simulink model "ConfiguredVirtualVehicleModelyaris"  (R2025b)
settings: configuration reference "VehicleVariable" (kept outside this file)
StartFcn:
  | %tic
StopFcn:
  | %toc
model workspace (MAT data in the model file):
  ExtDrvCmdsSwitch : Simulink.Parameter (value not decoded)
  ExtDrvRefSwitch : Simulink.Parameter (value not decoded)
  ExtEnvSwitch : Simulink.Parameter (value not decoded)
  ExtGndSwitch : Simulink.Parameter (value not decoded)
symbols that are objects in the model workspace (value not decoded): ExtDrvCmdsSwitch, ExtDrvRefSwitch, ExtEnvSwitch, ExtGndSwitch
undefined symbols (not defined in the file): AmbTemp, BaroPress, CurvGradRef, CurvRef, DCM, DriverAeroRes, DriverDrivelineRes, DriverInitialGear, DriverPreviewDist, DriverRollRes, DriverShiftTime, DriverTimeConst, DriverTractiveForce, EnvAbsPrs, EnvAirTemp, EnvGrvty, EnvNomFrictionScaling, EnvNominalGrade, EnvScnFrictionMap, EnvScnFrictionMapXBpts, EnvScnFrictionMapYBpts, EnvScnHeightMap, EnvScnHeightMapXBpts, EnvScnHeightMapYBpts, EnvWindVelX, EnvWindVelY, EnvWindVelZ, Gnd, Grade, HazzardCmd, HighBeamCmd, lambda_mux, LeftSignalCmd, LngRef, LowBeamCmd, LtrRef, PhiRef, PlntVehDstCGFrntAxl, PlntVehDstCGRearAxl, PlntVehInitLatPos, PlntVehInitLongPos, PlntVehInitPitchAng, PlntVehInitRollAng, PlntVehInitVertPos, PlntVehInitYawAng, PlntVehMass, PlntVehTrckWdth, PlntVehYawMomentInertia, PlntWhlLdRadiusFrnt, PlntWhlLdRadiusRear, RightSignalCmd, ScnCRRadius, Sim3dSensor, Wind, XRef, YRef, Z
libraries: simulink x28, autolibutils x8, autolibsharedcommon x7, vehdynlibscenariocommon x7, vehdynlibviscommon x4, vehdynlibdriver x2, sim3dgroundtruthsensorlib x2, sim3dlib x2, autolibshared x2, sim3dautolib x2, sl3dlib x1, sharedtransform x1
(part 3 of 6)

== system ConfiguredVirtualVehicleModelyaris/Visualization/External Output Routing ==
  VehFdbk : Inport
  Bus Assignment : BusAssignment  AssignedSignals=Driver.SteerFdbk,Driver.AccelFdbk,Driver.DecelFdbk,Driver.GearFdbk,Driver.IgnFdbk,Driveline.EngSpd,Driveline.TransGear,Body.InertFrm.Cg.Disp.X,Body.InertFrm.Cg.Disp.Y,Body.InertFrm.Cg.Disp.Z,Body.InertFrm.Cg.Vel.Xdot,Body.InertFrm.Cg.Vel.Ydot,Body.InertFrm.Cg.Vel.Zdot,Body.InertFrm.Cg.Ang.phi,Body.InertFrm.Cg.Ang.theta,Body.InertFrm.Cg.Ang.psi,Body.InertFrm.Geom.Disp.X,Body.InertFrm.Geom.Disp.Y,Body.InertFrm.Geom.Disp.Z,Body.InertFrm.Geom.Vel.Xdot,Body.InertFrm.Geom.Vel.Ydot,Body.InertFrm.Geom.Vel.Zdot,Body.BdyFrm.Cg.Vel.xdot,Body.BdyFrm.Cg.Vel.ydot,Body.BdyFrm.Cg.Vel.zdot,Body.BdyFrm.Cg.AngVel.p,Body.BdyFrm.Cg.AngVel.q,Body.BdyFrm.Cg.AngVel.r,Body.BdyFrm.Cg.Acc.ax,Body.BdyFrm.Cg.Acc.ay,Body.BdyFrm.Cg.Acc.az,Body.BdyFrm.Cg.Acc.xddot,Body.BdyFrm.Cg.Acc.yddot,Body.BdyFrm.Cg.Acc.zddot,Body.BdyFrm.Cg.AngAcc.pdot,Body.BdyFrm.Cg.AngAcc.qdot,Body.BdyFrm.Cg.AngAcc.rdot
  Bus Selector1 : BusSelector  OutputSignals=Driver.SteerFdbk,Driver.AccelFdbk,Driver.DecelFdbk,Driver.GearFdbk,Driver.IgnFdbk
  Bus Selector2 : BusSelector  OutputSignals=Body.InertFrm.Cg.Disp.X,Body.InertFrm.Cg.Disp.Y,Body.InertFrm.Cg.Disp.Z,Body.InertFrm.Cg.Vel.Xdot,Body.InertFrm.Cg.Vel.Ydot,Body.InertFrm.Cg.Vel.Zdot,Body.InertFrm.Cg.Ang.phi,Body.InertFrm.Cg.Ang.theta,Body.InertFrm.Cg.Ang.psi,Body.InertFrm.Geom.Disp.X,Body.InertFrm.Geom.Disp.Y,Body.InertFrm.Geom.Disp.Z,Body.InertFrm.Geom.Vel.Xdot,Body.InertFrm.Geom.Vel.Ydot,Body.InertFrm.Geom.Vel.Zdot,Body.BdyFrm.Cg.Vel.xdot,Body.BdyFrm.Cg.Vel.ydot,Body.BdyFrm.Cg.Vel.zdot,Body.BdyFrm.Cg.AngVel.p,Body.BdyFrm.Cg.AngVel.q,Body.BdyFrm.Cg.AngVel.r,Body.BdyFrm.Cg.Acc.ax,Body.BdyFrm.Cg.Acc.ay,Body.BdyFrm.Cg.Acc.az,Body.BdyFrm.Cg.Acc.xddot,Body.BdyFrm.Cg.Acc.yddot,Body.BdyFrm.Cg.Acc.zddot,Body.BdyFrm.Cg.AngAcc.pdot,Body.BdyFrm.Cg.AngAcc.qdot,Body.BdyFrm.Cg.AngAcc.rdot
  Bus Selector3 : BusSelector  OutputSignals=Engine.EngSpdOut,Trans.Info.Trans.TransGear
  Constant : Constant  Value=0  OutDataTypeStr=Bus: VVCVehFdbkBUS  SampleTime=-1
  Data Type Conversion : DataTypeConversion  SaturateOnIntegerOverflow=off  RndMeth=Floor
  Data Type Conversion1 : DataTypeConversion  SaturateOnIntegerOverflow=off  RndMeth=Floor
  Data Type Conversion2 : DataTypeConversion  SaturateOnIntegerOverflow=off  RndMeth=Floor
  Rate Transition : RateTransition  Integrity=off
  Rate Transition1 : RateTransition  Integrity=off
  Rate Transition2 : RateTransition  Integrity=off
  Unit Conversion{1..8} (8 alike) : UnitConversion
  ExtVehFdbk : Outport
  wires:
  Constant/1 -> Bus Assignment/1
  Bus Assignment/1 -> ExtVehFdbk/1
  Bus Selector1/1 -> Unit Conversion2/1  "<SteerFdbk>"
  Bus Selector1/2 -> Bus Assignment/3  "<AccelFdbk>"
  Bus Selector1/3 -> Bus Assignment/4  "<DecelFdbk>"
  Bus Selector1/4 -> Data Type Conversion1/1  "<GearFdbk>"
  Bus Selector1/5 -> Data Type Conversion2/1  "<IgnFdbk>"
  Bus Selector3/1 -> Unit Conversion1/1  "<EngSpdOut>"
  Bus Selector3/2 -> Data Type Conversion/1  "<TransGear>"
  Data Type Conversion/1 -> Bus Assignment/8
  Data Type Conversion1/1 -> Bus Assignment/5
  Data Type Conversion2/1 -> Bus Assignment/6
  Unit Conversion1/1 -> Bus Assignment/7
  Unit Conversion2/1 -> Bus Assignment/2
  Bus Selector2/1 -> Bus Assignment/9  "<X>"
  Bus Selector2/2 -> Bus Assignment/10  "<Y>"
  Bus Selector2/3 -> Bus Assignment/11  "<Z>"
  Bus Selector2/4 -> Bus Assignment/12  "<Xdot>"
  Bus Selector2/5 -> Bus Assignment/13  "<Ydot>"
  Bus Selector2/6 -> Bus Assignment/14  "<Zdot>"
  Bus Selector2/7 -> Unit Conversion6/1  "<phi>"
  Bus Selector2/8 -> Unit Conversion7/1  "<theta>"
  Bus Selector2/9 -> Unit Conversion8/1  "<psi>"
  Bus Selector2/10 -> Bus Assignment/18  "<X>"
  Bus Selector2/11 -> Bus Assignment/19  "<Y>"
  Bus Selector2/12 -> Bus Assignment/20  "<Z>"
  Bus Selector2/13 -> Bus Assignment/21  "<Xdot>"
  Bus Selector2/14 -> Bus Assignment/22  "<Ydot>"
  Bus Selector2/15 -> Bus Assignment/23  "<Zdot>"
  Bus Selector2/16 -> Bus Assignment/24  "<xdot>"
  Bus Selector2/17 -> Bus Assignment/25  "<ydot>"
  Bus Selector2/18 -> Bus Assignment/26  "<zdot>"
  Bus Selector2/19 -> Bus Assignment/27  "<p>"
  Bus Selector2/20 -> Bus Assignment/28  "<q>"
  Bus Selector2/21 -> Bus Assignment/29  "<r>"
  Bus Selector2/22 -> Unit Conversion3/1  "<ax>"
  Bus Selector2/23 -> Unit Conversion4/1  "<ay>"
  Bus Selector2/24 -> Unit Conversion5/1  "<az>"
  Bus Selector2/25 -> Bus Assignment/33  "<xddot>"
  Bus Selector2/26 -> Bus Assignment/34  "<yddot>"
  Bus Selector2/27 -> Bus Assignment/35  "<zddot>"
  Bus Selector2/28 -> Bus Assignment/36  "<pdot>"
  Bus Selector2/29 -> Bus Assignment/37  "<qdot>"
  Bus Selector2/30 -> Bus Assignment/38  "<rdot>"
  Unit Conversion3/1 -> Bus Assignment/30
  Unit Conversion4/1 -> Bus Assignment/31
  Unit Conversion5/1 -> Bus Assignment/32
  Unit Conversion6/1 -> Bus Assignment/15
  Unit Conversion7/1 -> Bus Assignment/16
  Unit Conversion8/1 -> Bus Assignment/17
  VehFdbk/1 -> Rate Transition/1, Rate Transition2/1, Rate Transition1/1
  Rate Transition/1 -> Bus Selector1/1
  Rate Transition1/1 -> Bus Selector3/1
  Rate Transition2/1 -> Bus Selector2/1

== system ConfiguredVirtualVehicleModelyaris/Visualization/ISO 15037-1:2006 ==
  VehFdbk : Inport
  Disabled : Subsystem  VariantControl=0
  Enabled : Subsystem  VariantControl=1

== system ConfiguredVirtualVehicleModelyaris/Visualization/Performance Calculations ==
  VehSpd : Inport
  FuelVolFlow : Inport  Port=2
  BattPwr : Inport  Port=3
  Add : Sum
  Divide : Product  Inputs=*/
  Divide1 : Product  Inputs=*/
  Divide2 : Product  Inputs=*/
  Integrator : Integrator
  Integrator1 : Integrator
  L/100 Km Calc : Product  Inputs=/*
  Product : Product
  Rate Transition3 : RateTransition  Deterministic=off
  Saturation : Saturate  UpperLimit=Inf  LowerLimit=0.001  ZeroCross=off
  Saturation1 : Saturate  UpperLimit=Inf  LowerLimit=1e-3  ZeroCross=off
  Signal Specification5 : SignalSpecification  Unit=m/s
  Sqrt : Sqrt
  US EPA kwh/USgal equivalent : Constant  Value=33.7
  US MPG Calc : Product  Inputs=*/
  Unit Conversion5 : UnitConversion
  m to 100Km : Gain  Gain=1/1000/100
  m to mile : Gain  Gain=0.000621371
  m^3 per gal : Gain  Gain=0.00378541
  m^3 to L : Gain  Gain=1000
  m^3 to US Gal : Gain  Gain=264.172
  s per h : Constant  Value=3600
  w per kw : Constant  Value=1000
  US MPG : Outport  VectorParamsAs1DForOutWhenUnconnected=off
  L/100Km : Outport  Port=2  VectorParamsAs1DForOutWhenUnconnected=off
  wires:
  m^3 to US Gal/1 -> Saturation1/1
  m^3 to L/1 -> L/100 Km Calc/2
  Integrator/1 -> m to mile/1, m to 100Km/1
  m to mile/1 -> US MPG Calc/1
  FuelVolFlow/1 -> Add/1
  Integrator1/1 -> m^3 to US Gal/1, m^3 to L/1
  Saturation/1 -> L/100 Km Calc/1
  m to 100Km/1 -> Saturation/1
  L/100 Km Calc/1 -> L/100Km/1  "L/100Km"
  US MPG Calc/1 -> Rate Transition3/1
  Saturation1/1 -> US MPG Calc/2
  Rate Transition3/1 -> US MPG/1  "US MPG"
  w per kw/1 -> Divide/2
  Divide/1 -> Divide2/1
  Divide2/1 -> Divide1/1
  s per h/1 -> Divide1/2
  Divide1/1 -> m^3 per gal/1
  Add/1 -> Integrator1/1
  m^3 per gal/1 -> Add/2
  US EPA kwh/USgal equivalent/1 -> Divide2/2
  BattPwr/1 -> Divide/1
  Sqrt/1 -> Integrator/1
  Product/1 -> Sqrt/1
  Signal Specification5/1 -> Product/2, Product/1
  Unit Conversion5/1 -> Signal Specification5/1
  VehSpd/1 -> Unit Conversion5/1

== system ConfiguredVirtualVehicleModelyaris/Visualization/Scope Type ==
  "VehFdbk " : Inport
  "Vis " : Inport  Port=2
  DLC : Subsystem  VariantControl=1
  None : Subsystem  VariantControl=0
  XYZ : Subsystem  VariantControl=2
  " Ref" : Outport  VectorParamsAs1DForOutWhenUnconnected=off

== system ConfiguredVirtualVehicleModelyaris/Visualization/Vehicle XY Plotter ==
  "VehFdbk " : Inport
  "Ref " : Inport  Port=2
  Disabled : Subsystem  VariantControl=2
  XY View : Subsystem  VariantControl=0
  XY View Ref : Subsystem  VariantControl=1
  XY View Ref with One-Axle Trailer : Subsystem  VariantControl=3

== system ConfiguredVirtualVehicleModelyaris/Driver Commands/Driver Commands/Dashboard Widgets ==
  note: Controls
  VehFdbk : Inport
  Hazards : LampBlock  LabelPosition=Hide  DefaultColor=[192.0, 192.0, 192.0]  Icon=Hazards
  High Beams : LampBlock  LabelPosition=Hide  DefaultColor=[192.0, 192.0, 192.0]  Icon=HighBeams
  Knob : KnobBlock  LabelPosition=Bottom  ScaleMin=-90  ScaleMax=90  TickInterval=30
  Low Beams : LampBlock  LabelPosition=Hide  DefaultColor=[192.0, 192.0, 192.0]  Icon=LowBeams
  Push Button : PushButtonBlock  ButtonText=Hazzard  ButtonType=Latch  Icon=Hazards  IconOnColor=[1.0, 0.0, 0.0]  IconOffColor=[0.50196078431372548, 0.50196078431372548, 0.50196078431372548]  IconColor=On  OffValue=0.000000
  Push Button1 : PushButtonBlock  ButtonText=Start / Stop  ButtonType=Latch  IconOnColor=[0.0, 1.0, 0.0]  IconOffColor=[0.0, 0.0, 0.0]  IconColor=On  OffValue=0.000000
  Rotary Switch : RotarySwitchBlock  LabelPosition=Bottom
  Rotary Switch1 : RotarySwitchBlock  LabelPosition=Bottom
  Rotary Switch2 : RotarySwitchBlock  LabelPosition=Bottom
  Slider : SliderBlock  LabelPosition=Bottom  ScaleMax=1  TickInterval=.2
  Slider1 : SliderBlock  LabelPosition=Bottom  ScaleMax=1  TickInterval=.2
  Turn Signal Left : LampBlock  LabelPosition=Hide  DefaultColor=[192.0, 192.0, 192.0]  Icon=TurnSignalLeft
  Turn Signal Right : LampBlock  LabelPosition=Hide  DefaultColor=[192.0, 192.0, 192.0]  Icon=TurnSignalRight
  Widget Sinks : Subsystem
  Widget Sources : Subsystem
  Driver : Outport  VectorParamsAs1DForOutWhenUnconnected=off
  wires:
  VehFdbk/1 -> Widget Sinks/1(VehFdbk)
  Widget Sources/1(Driver) -> Driver/1

== system ConfiguredVirtualVehicleModelyaris/Driver Commands/Driver Commands/Game Wheel Hardware ==
  VehFdbk : Inport
  Add : Sum  Inputs=-+
  Bus Creator1 : BusCreator  Inputs=6
  Compare To Zero : simulink/Logic and Bit Operations/Compare To Zero  relop=~=  OutDataTypeStr=boolean
  Constant : Constant  Value=false
  Constant1 : Constant
  Constant2 : Constant
  Cont LPF : autolibutils/Cont LPF  wc=10*2*pi  AbsoluteTolerance=auto  aMode=6
  Cont LPF1 : autolibutils/Cont LPF  wc=10*2*pi  AbsoluteTolerance=auto  aMode=6
  Dead Zone : DeadZone  LowerValue=0  UpperValue=.01  ZeroCross=off
  Demux1 : Demux  Outputs=2
  Gain : Gain  Gain=.5
  Game Wheel Input Requires Simulink 3D Animation Signal dimensions and scaling are hardware dependent : sl3dlib/Simulation 3D/Hardware Interface/Simulation 3D Joystick  Commented=on  joyid=1  adjustports=off  forcefeed=off
  Manual Switch : ManualSwitch  CurrentSetting=0
  OR : Logic  Operator=OR  IconShape=distinctive  AllPortsSameDT=off  OutDataTypeStr=boolean
  Paddle Shift : Subsystem
  Selector : Selector  InputPortWidth=8  IndexOptions=Index vector (dialog)  Indices=[1]  OutputSizes=1
  Selector1 : Selector  InputPortWidth=8  IndexOptions=Index vector (dialog)  Indices=[2 3]  OutputSizes=1
  Signal Specification : SignalSpecification  Unit=1
  Signal Specification1 : SignalSpecification  Unit=1
  Signal Specification2 : SignalSpecification  Unit=1
  Signal Specification3 : SignalSpecification  Unit=rad
  Stick Shift : Subsystem
  Switch : Switch  Criteria=u2 ~= 0  SaturateOnIntegerOverflow=off  InputSameDT=off
  Terminator : Terminator
  To Virtual Bus : SignalConversion  ConversionOutput=Virtual bus  OverrideOpt=off
  Unit Delay : UnitDelay  SampleTime=-1  HasFrameUpgradeWarning=on
  VVCLightsCmd : Constant  Value=0  OutDataTypeStr=Bus: VVCLightsCmdBUS  SampleTime=-1
  Wheel Angle Limit [rad] : Gain  Gain=2*2*pi
  Driver : Outport  VectorParamsAs1DForOutWhenUnconnected=off
  wires:
  Stick Shift/1(Gear) -> Manual Switch/2
  Paddle Shift/1(Gear) -> Manual Switch/1
  Game Wheel Input Requires Simulink 3D Animation Signal dimensions and scaling are hardware dependent/2 -> Paddle Shift/1(Buttons), Stick Shift/1(Buttons)
  Game Wheel Input Requires Simulink 3D Animation Signal dimensions and scaling are hardware dependent/1 -> Selector/1, Selector1/1
  To Virtual Bus/1 -> Bus Creator1/6  "LightsCmd"
  VVCLightsCmd/1 -> To Virtual Bus/1
  Constant1/1 -> Add/2
  Cont LPF/1 -> Wheel Angle Limit [rad]/1
  Demux1/1 -> Signal Specification/1
  Cont LPF1/1 -> Dead Zone/1
  Manual Switch/1 -> Signal Specification2/1
  Wheel Angle Limit [rad]/1 -> Signal Specification3/1
  Demux1/2 -> Signal Specification1/1
  Add/1 -> Gain/1
  Selector/1 -> Cont LPF/1
  Dead Zone/1 -> Demux1/1
  Gain/1 -> Cont LPF1/1
  Constant/1 -> Bus Creator1/5  "IgnSwtch"
  Signal Specification1/1 -> Bus Creator1/3  "DecelCmd"
  Signal Specification/1 -> Bus Creator1/2  "AccelCmd"
  VehFdbk/1 -> Terminator/1
  Bus Creator1/1 -> Driver/1
  Signal Specification3/1 -> Bus Creator1/1  "SteerCmd"
  Signal Specification2/1 -> Bus Creator1/4  "GearCmd"
  OR/1 -> Unit Delay/1, Switch/2
  Selector1/1 -> Switch/1, Compare To Zero/1
  Compare To Zero/1 -> OR/1
  Unit Delay/1 -> OR/2
  Switch/1 -> Add/1
  Constant2/1 -> Switch/3

== system ConfiguredVirtualVehicleModelyaris/Driver Commands/Driver Commands/Longitudinal Driver ==
  VehRef : Inport
  VehFdbk : Inport  Port=2
  Env : Inport  Port=3
  Bus Creator1 : BusCreator  Inputs=6
  Bus Selector1 : BusSelector  OutputSignals=DrvCmd.SteerCmd.SteerCmd,DrvRef.LngRef,DrvCmd.AccelCmd.EnblAccelCmd,DrvCmd.AccelCmd.AccelCmd,DrvCmd.AccelCmd.AccelHld,DrvCmd.AccelCmd.AccelZero,DrvCmd.DecelCmd.EnblDecelCmd,DrvCmd.DecelCmd.DecelCmd,DrvCmd.DecelCmd.DecelHld,DrvCmd.DecelCmd.DecelZero
  Constant : Constant  Value=false
  Hill Hold & Stop : Subsystem
  Longitudinal Driver : Subsystem  SystemSampleTime=.01  mask(Longitudinal Driver){extAccelOvr=on, extDecelOvr=on, extAccelHld=on, extDecelHld=on, extAccelZero=on, extDecelZero=on, cntrlType=Predictive, shftType=Reverse, Neutral, Drive, velUnits=m/s, gearOut=on, Kp=10, Ki=5, Kff=.1, Kg=0, VehVelVec=[0 100], KffVec=[.1 .1], KpVec=[10 10], KiVec=[5 5], KgVec=[0 0], m=PlntVehMass, Kpt=DriverTractiveForce, tau=DriverTimeConst, L=DriverPreviewDist, aR=DriverRollRes, bR=DriverDrivelineRes, cR=DriverAeroRes, g=EnvGrvty, vnom=5, Kaw=1, tauerr=.01, tauPt=2, GearInit=DriverInitialGear, tShift=DriverShiftTime, pdlVec=[0.1 0.4 0.5 0.9], upShftTbl=[-1 12.9375 26.4375 39.9375 51.18749999999999 62.4375 72.84375 83.25;-1 16.3125 29.8125 43.3125 54.5624 65.8125 76.78125 87.75;-1 19.6875 33.1875 46.68749999999999 57.9375 69.1875 80.71875 92.25;-1 33 52.5 77.25 100.5 138.75 161.875 185], dwnShftTbl=[1 9.5625 23.0625 36.5625 47.8125 59.0625 68.90625 78.75;1 12.9375 26.4375 39.9375 51.18749999999999 62.4375 72.84375 83.25;1 16.3125 29.8125 43.3125 54.562499 65.8125 76.78125 87.75;1 19.6875 33.1875 46.68749999999999 57.9375 69.1875 80.71875 92.25], tClutch=.5, tRev=.5, tPark=120, aMode=6, UpGearVec=[0  1  2  3  4  5  6  7], DownGearVec=[1  2  3  4  5  6  7  8]}
      mask prompts: extAccelOvr "autoblks_shared:autoblkLongitudinalDriver:blkPrm_extAccelOvr"; extDecelOvr "autoblks_shared:autoblkLongitudinalDriver:blkPrm_extDeccelOvr"; extAccelHld "autoblks_shared:autoblkLongitudinalDriver:blkPrm_extAccelHld"; extDecelHld "autoblks_shared:autoblkLongitudinalDriver:blkPrm_extDeccelHld"; extAccelZero "autoblks_shared:autoblkLongitudinalDriver:blkPrm_extAccelZero"; extDecelZero "autoblks_shared:autoblkLongitudinalDriver:blkPrm_extDeccelZero"; cntrlType "autoblks_shared:autoblkLongitudinalDriver:blkPrm_cntrlType"; shftType "autoblks_shared:autoblkLongitudinalDriver:blkPrm_shftType"; velUnits "autoblks_shared:autoblkLongitudinalDriver:blkPrm_velUnits"; gearOut "autoblks_shared:autoblkLongitudinalDriver:blkPrm_gearOut"; Kp "autoblks_shared:autoblkLongitudinalDriver:blkPrm_Kp"; Ki "autoblks_shared:autoblkLongitudinalDriver:blkPrm_Ki"; Kff "autoblks_shared:autoblkLongitudinalDriver:blkPrm_Kff"; Kg "autoblks_shared:autoblkLongitudinalDriver:blkPrm_Kg"; VehVelVec "autoblks_shared:autoblkLongitudinalDriver:blkPrm_VehVelVec"; KffVec "autoblks_shared:autoblkLongitudinalDriver:blkPrm_KffVec"; KpVec "autoblks_shared:autoblkLongitudinalDriver:blkPrm_KpVec"; KiVec "autoblks_shared:autoblkLongitudinalDriver:blkPrm_KiVec"; KgVec "autoblks_shared:autoblkLongitudinalDriver:blkPrm_KgVec"; m "autoblks_shared:autoblkLongitudinalDriver:blkPrm_m"; Kpt "autoblks_shared:autoblkLongitudinalDriver:blkPrm_Kpt"; tau "autoblks_shared:autoblkLongitudinalDriver:blkPrm_tau"; L "autoblks_shared:autoblkLongitudinalDriver:blkPrm_L"; aR "autoblks_shared:autoblkLongitudinalDriver:blkPrm_aR"; bR "autoblks_shared:autoblkLongitudinalDriver:blkPrm_bR"; cR "autoblks_shared:autoblkLongitudinalDriver:blkPrm_cR"; g "autoblks_shared:autoblkLongitudinalDriver:blkPrm_g"; vnom "autoblks_shared:autoblkLongitudinalDriver:blkPrm_vnom"; Kaw "autoblks_shared:autoblkLongitudinalDriver:blkPrm_Kaw"; tauerr "autoblks_shared:autoblkLongitudinalDriver:blkPrm_tauerr"; tauPt "autoblks_shared:autoblkLongitudinalDriver:blkPrm_tauPt"; GearInit "autoblks_shared:autoblkLongitudinalDriver:blkPrm_GearInit"; tShift "autoblks_shared:autoblkLongitudinalDriver:blkPrm_tShift"; pdlVec "autoblks_shared:autoblkLongitudinalDriver:blkPrm_pdlVec"; upShftTbl "autoblks_shared:autoblkLongitudinalDriver:blkPrm_upShftTbl"; dwnShftTbl "autoblks_shared:autoblkLongitudinalDriver:blkPrm_dwnShftTbl"; tClutch "autoblks_shared:autoblkLongitudinalDriver:blkPrm_tClutch"; tRev "autoblks_shared:autoblkLongitudinalDriver:blkPrm_tRev"; tPark "autoblks_shared:autoblkLongitudinalDriver:blkPrm_tPark"; UpGearVec "autoblks_shared:autoblkLongitudinalDriver:blkPrm_UpGearVec"; DownGearVec "autoblks_shared:autoblkLongitudinalDriver:blkPrm_DownGearVec"
      mask help: autoblks_shared:autoblkLongitudinalDriver:blkDesc
      mask init:
      | [~]=autosharedicon('autoliboperlong',gcb,0);
      mask Help: eval('autosharedhelp(''pbopmodlong'')');
      mask TypeOptions cntrlType: autoblks_shared:autoblkLongitudinalDriver:blkCmb_cntrlType_c1 | autoblks_shared:autoblkLongitudinalDriver:blkCmb_cntrlType_c2 | autoblks_shared:autoblkLongitudinalDriver:blkCmb_cntrlType_c3
      mask Callback cntrlType: [~]=autosharedicon('autoliboperlong',gcb,1);
      mask TypeOptions shftType: Longitudinal Driver/shftType
      mask Callback shftType: [~]=autosharedicon('autoliboperlong',gcb,1);
      mask TypeOptions velUnits: VelRef/Unit
      mask Callback velUnits: [~]=autosharedicon('autoliboperlong',gcb,1);
      mask DialogControl modeConfig Prompt: autoblks_shared:autoblkLongitudinalDriver:blkDlg_modeConfig
      mask DialogControl sigConfigPanel Prompt: autoblks_shared:autoblkLongitudinalDriver:blkDlg_sigConfigPanel
      mask DialogControl extAccelOvr Prompt: Accelerator override
      mask DialogControl extDecelOvr Prompt: Decelerator override
      mask DialogControl extAccelHld Prompt: Accelerator hold
      mask DialogControl extDecelHld Prompt: Decelerator hold
      mask DialogControl extAccelZero Prompt: Accelerator disable
      mask DialogControl extDecelZero Prompt: Decelerator disable
      mask DialogControl cntrlType Prompt: Control type, cntrlType:
      mask DialogControl shftType Prompt: Shift type, shftType:
      mask DialogControl velUnits Prompt: Reference and feedback units, velUnits [velUnits]:
      mask DialogControl gearOut Prompt: Output gear signal
      mask DialogControl CntrlParamPanel Prompt: autoblks_shared:autoblkLongitudinalDriver:blkDlg_CntrlParamPanel
      mask DialogControl PIParam Prompt: autoblks_shared:autoblkLongitudinalDriver:blkDlg_PIParam
      mask DialogControl Kp Prompt: Proportional gain, Kp []:
      mask DialogControl Ki Prompt: Integral gain, Ki []:
      mask DialogControl Kff Prompt: Velocity feed-forward, Kff []:
      mask DialogControl Kg Prompt: Grade angle feed-forward, Kg [1/deg]:
      mask DialogControl PISchedParam Prompt: autoblks_shared:autoblkLongitudinalDriver:blkDlg_PISchedParam
      mask DialogControl VehVelVec Prompt: Velocity gain breakpoints:
      mask DialogControl KffVec Prompt: Velocity feed-forward gain values, KffVec []:
      mask DialogControl KpVec Prompt: Proportional gain values, KpVec []:
      mask DialogControl KiVec Prompt: Integral gain values, KiVec []:
      mask DialogControl KgVec Prompt: Grade angle feed-forward values, KgVec [1/deg]:
      mask DialogControl PredParam Prompt: autoblks_shared:autoblkLongitudinalDriver:blkDlg_PredParam
      mask DialogControl m Prompt: Vehicle mass, m [kg]:
      mask DialogControl Kpt Prompt: Effective vehicle total tractive force, Kpt [N]:
      mask DialogControl tau Prompt: Driver response time, tau [s]:
      mask DialogControl L Prompt: Preview distance, L [m]:
      mask DialogControl aR Prompt: Rolling resistance coefficient, aR [N]:
      mask DialogControl bR Prompt: Rolling and driveline resistance coefficient, bR [N*s/m]:
      mask DialogControl cR Prompt: Aerodynamic drag coefficient, cR [N*s^2/m^2]:
      mask DialogControl g Prompt: Gravitational constant, g [m/s^2]:
      mask DialogControl vnom Prompt: Nominal speed, vnom [velUnits]:
      mask DialogControl Kaw Prompt: Anti-windup, Kaw []:
      mask DialogControl tauerr Prompt: Error filter time constant, tauerr [s]:
      mask DialogControl tauPt Prompt: Powertrain time constant, tauPt [s]:
      mask DialogControl shiftParamPanel Prompt: autoblks_shared:autoblkLongitudinalDriver:blkDlg_shiftParamPanel
      mask DialogControl GearInit Prompt: Initial gear, GearInit []:
      mask DialogControl tShift Prompt: Time required to shift, tShift [s]:
      mask DialogControl pdlVec Prompt: Up and down shift accelerator pedal positions, pdlVec []:
      mask DialogControl upShftTbl Prompt: Upshift velocity data table, upShftTbl [velUnits]:
      mask DialogControl dwnShftTbl Prompt: Downshift velocity data table, dwnShftTbl [velUnits]:
      mask DialogControl tClutch Prompt: Time required to shift, tClutch [s]:
      mask DialogControl tRev Prompt: Time required to engage reverse from neutral, tRev [s]:
      mask DialogControl tPark Prompt: Time required to engage park from neutral, tPark [s]:
      mask DialogControl UpGearVec Prompt: Upshift gear vector, UpGearVec []:
      mask DialogControl DownGearVec Prompt: Downshift gear vector, DownGearVec []:
      mask Display:
      | try
      |     IconInfo = autosharedicon('autoliboperlong', gcb, 4);
      | 
      |     image(IconInfo.image, IconInfo.position);
      | 
      |     for i = 1:numel(IconInfo.lconn)
      |         port_label('lconn', i, IconInfo.lconn{i})
      |     end
      | 
      |     for j = 1:numel(IconInfo.rconn)
      |         port_label('rconn', j, IconInfo.rconn{j})
      |     end
      | 
      |     for k = 1:numel(IconInfo.input)
      |         port_label('input', k, IconInfo.input{k})
      |     end
      | 
      |     for m = 1:numel(IconInfo.output)
      |         port_label('output', m, IconInfo.output{m})
      |     end
      | catch
      |     fprintf('Longitudinal \n Driver')
      | end
  Signal Specification : SignalSpecification  Unit=rad
  Terminator3 : Terminator
  To Nonvirtual Bus : SignalConversion  ConversionOutput=Virtual bus  OverrideOpt=off
  Unit Conversion : UnitConversion
  Unit Conversion1 : UnitConversion
  VVCLightsCmd : Constant  Value=0  OutDataTypeStr=Bus: VVCLightsCmdBUS  SampleTime=-1
  Driver : Outport  VectorParamsAs1DForOutWhenUnconnected=off
  wires:
  Signal Specification/1 -> Bus Creator1/1  "SteerCmd"
  To Nonvirtual Bus/1 -> Bus Creator1/6  "LightsCmd"
  VVCLightsCmd/1 -> To Nonvirtual Bus/1
  Hill Hold & Stop/6(Grade) -> Longitudinal Driver/11(Grade)
  Hill Hold & Stop/5(VelFdbk) -> Longitudinal Driver/10(VelFdbk)
  Bus Selector1/5 -> Longitudinal Driver/4(AccelHld)  "<AccelHld>"
  Unit Conversion1/1 -> Longitudinal Driver/1(VelRef), Hill Hold & Stop/1(LngRef)
  Hill Hold & Stop/4(DecelZero) -> Longitudinal Driver/9(DecelZero)
  Hill Hold & Stop/3(DecelHld) -> Longitudinal Driver/8(DecelHld)
  Env/1 -> Hill Hold & Stop/6(Env)
  Hill Hold & Stop/1(EnblDecelOvr) -> Longitudinal Driver/6(EnblDecelOvr)
  Hill Hold & Stop/2(DecelOvrCmd) -> Longitudinal Driver/7(DecelOvrCmd)
  Bus Selector1/10 -> Hill Hold & Stop/5(<DecelZero>)  "<DecelZero>"
  Bus Selector1/9 -> Hill Hold & Stop/4(<DecelHld>)  "<DecelHld>"
  Bus Selector1/8 -> Hill Hold & Stop/3(<DecelOvrCmd>)  "<DecelCmd>"
  Bus Selector1/7 -> Hill Hold & Stop/2(<EnblDecelCmd>)  "<EnblDecelCmd>"
  Bus Selector1/6 -> Longitudinal Driver/5(AccelZero)  "<AccelZero>"
  Bus Selector1/4 -> Longitudinal Driver/3(AccelOvrCmd)  "<AccelCmd>"
  Bus Selector1/3 -> Longitudinal Driver/2(EnblAccelOvr)  "<EnblAccelCmd>"
  Constant/1 -> Bus Creator1/5  "IgnSwtch"
  Bus Selector1/1 -> Unit Conversion/1  "<SteerCmd>"
  Longitudinal Driver/4(GearCmd) -> Bus Creator1/4  "GearCmd"
  Longitudinal Driver/2(AccelCmd) -> Bus Creator1/2  "AccelCmd"
  VehFdbk/1 -> Hill Hold & Stop/7(VehFdbk)
  VehRef/1 -> Bus Selector1/1
  Bus Selector1/2 -> Unit Conversion1/1  "<LngRef>"
  Longitudinal Driver/1(Info) -> Terminator3/1
  Longitudinal Driver/3(DecelCmd) -> Bus Creator1/3  "DecelCmd"
  Unit Conversion/1 -> Signal Specification/1
  Bus Creator1/1 -> Driver/1

== system ConfiguredVirtualVehicleModelyaris/Driver Commands/Driver Commands/No Driver ==
  VehRef : Inport
  VehFdbk : Inport  Port=2
  Env : Inport  Port=3
  Bus Creator1 : BusCreator  Inputs=6
  Bus Selector1 : BusSelector  OutputSignals=DrvCmd.SteerCmd.SteerCmd,DrvCmd.AccelCmd.AccelCmd,DrvCmd.DecelCmd.DecelCmd,DrvCmd.TransCmd.GearCmd,DrvCmd.IgnModeCmd,DrvCmd.LightsCmd
  Data Type Conversion : DataTypeConversion  SaturateOnIntegerOverflow=off  RndMeth=Floor
  Data Type Conversion1 : DataTypeConversion  SaturateOnIntegerOverflow=off  RndMeth=Floor
  Signal Specification{,1..3} (4 alike) : SignalSpecification  Unit=1
  Signal Specification4 : SignalSpecification  Unit=rad
  Terminator : Terminator
  Terminator1 : Terminator
  To Nonvirtual Bus : SignalConversion  ConversionOutput=Virtual bus  OverrideOpt=off
  Unit Conversion{,1..3} (4 alike) : UnitConversion
  Driver : Outport  VectorParamsAs1DForOutWhenUnconnected=off
  wires:
  Unit Conversion/1 -> Signal Specification4/1
  Data Type Conversion/1 -> Signal Specification3/1
  Unit Conversion3/1 -> Signal Specification2/1
  Unit Conversion2/1 -> Signal Specification1/1
  Unit Conversion1/1 -> Signal Specification/1
  Data Type Conversion1/1 -> Unit Conversion3/1
  Bus Selector1/5 -> Data Type Conversion/1  "<IgnModeCmd>"
  Bus Selector1/6 -> To Nonvirtual Bus/1  "<LightsCmd>"
  Bus Selector1/4 -> Data Type Conversion1/1  "<GearCmd>"
  Bus Selector1/3 -> Unit Conversion2/1  "<DecelCmd>"
  To Nonvirtual Bus/1 -> Bus Creator1/6  "LightsCmd"
  Env/1 -> Terminator1/1
  Signal Specification3/1 -> Bus Creator1/5  "IgnSwtch"
  Bus Selector1/1 -> Unit Conversion/1  "<SteerCmd>"
  Signal Specification2/1 -> Bus Creator1/4  "GearCmd"
  Signal Specification/1 -> Bus Creator1/2  "AccelCmd"
  VehFdbk/1 -> Terminator/1
  VehRef/1 -> Bus Selector1/1
  Bus Selector1/2 -> Unit Conversion1/1  "<AccelCmd>"
  Signal Specification1/1 -> Bus Creator1/3  "DecelCmd"
  Signal Specification4/1 -> Bus Creator1/1  "SteerCmd"
  Bus Creator1/1 -> Driver/1

== system ConfiguredVirtualVehicleModelyaris/Driver Commands/Driver Commands/Open Loop ==
  VehFdbk : Inport
  SteerCmd : Inport  Port=2
  AccelCmd : Inport  Port=3
  BrakeCmd : Inport  Port=4
  GearCmd : Inport  Port=5
  Bus Creator1 : BusCreator  Inputs=6
  Constant : Constant  Value=false
  Signal Specification : SignalSpecification  Unit=1
  Signal Specification1 : SignalSpecification  Unit=1
  Signal Specification2 : SignalSpecification  Unit=1
  Terminator : Terminator
  To Nonvirtual Bus : SignalConversion  ConversionOutput=Virtual bus  OverrideOpt=off
  Unit Conversion : UnitConversion
  VVCLightsCmd : Constant  Value=0  OutDataTypeStr=Bus: VVCLightsCmdBUS  SampleTime=-1
  Wheel Angle Limit * Steer Ratio : Gain  Gain=40*pi/180*18
  Driver : Outport  VectorParamsAs1DForOutWhenUnconnected=off
  wires:
  To Nonvirtual Bus/1 -> Bus Creator1/6  "LightsCmd"
  VVCLightsCmd/1 -> To Nonvirtual Bus/1
  Constant/1 -> Bus Creator1/5  "IgnSwtch"
  Signal Specification1/1 -> Bus Creator1/3  "DecelCmd"
  GearCmd/1 -> Signal Specification2/1
  Signal Specification/1 -> Bus Creator1/2  "AccelCmd"
  SteerCmd/1 -> Unit Conversion/1
  VehFdbk/1 -> Terminator/1
  AccelCmd/1 -> Signal Specification/1
  Unit Conversion/1 -> Wheel Angle Limit * Steer Ratio/1
  Bus Creator1/1 -> Driver/1
  Wheel Angle Limit * Steer Ratio/1 -> Bus Creator1/1  "SteerCmd"
  BrakeCmd/1 -> Signal Specification1/1
  Signal Specification2/1 -> Bus Creator1/4  "GearCmd"

== system ConfiguredVirtualVehicleModelyaris/Driver Commands/Driver Commands/Predictive Driver ==
  VehRef : Inport
  VehFdbk : Inport  Port=2
  Env : Inport  Port=3
  Bus Creator1 : BusCreator  Inputs=6
  Bus Selector : BusSelector  OutputSignals=Body.InertFrm.Cg.Disp.Y,Body.InertFrm.Cg.Vel.Ydot,Body.InertFrm.Cg.Ang.psi,Body.BdyFrm.Cg.AngVel.r
  Bus Selector1 : BusSelector  OutputSignals=DrvRef.LngRef,DrvRef.LtrRef,DrvCmd.SteerCmd.EnblSteerCmd,DrvCmd.SteerCmd.SteerCmd,DrvCmd.SteerCmd.SteerHld,DrvCmd.SteerCmd.SteerZero,DrvCmd.AccelCmd.EnblAccelCmd,DrvCmd.AccelCmd.AccelCmd,DrvCmd.AccelCmd.AccelHld,DrvCmd.AccelCmd.AccelZero,DrvCmd.DecelCmd.EnblDecelCmd,DrvCmd.DecelCmd.DecelCmd,DrvCmd.DecelCmd.DecelHld,DrvCmd.DecelCmd.DecelZero
  Constant : Constant  Value=false
  Hill Hold & Stop : Subsystem
  Linear Predictive Driver : vehdynlibdriver/Predictive Driver  extAccelOvr=on  extDecelOvr=on  extAccelHld=on  extDecelHld=on  extAccelZero=on  extDecelZero=on  extSteerOvr=on  extSteerHld=on  extSteerZero=on  cntrlType=Predictive  cntrlTypeLat=Predictive  shftType=Reverse, Neutral, Drive  coordMode=SAE J670 (Z-down)  refType=Reference pose  velUnits=m/s  angUnits=rad  gearOut=on  steerOut=on  Kp=3  Ki=1  Kff=1  Kg=0  VehVelVec=[0 100]  KffVec=[.1 .1]  KpVec=[10 10]  KiVec=[5 5]  KgVec=[0 0]  vnom=5  Kaw=1  tauerr=.075  tau=DriverTimeConst  L=DriverPreviewDist  Kpt=DriverTractiveForce  aR=DriverRollRes  bR=DriverDrivelineRes  cR=DriverAeroRes  g=EnvGrvty  vecPose=off  dynamMode=off  PositionGainF=2.5  PositionGainR=2.5  YawRateGain=.2  DelayGain=.2  enableDrift=off  BetaRef=10  KpBeta=1  KpDrift=1  KdDrift=1  KpPsi=1  KOmega=.1  tOmega=.1  a=PlntVehDstCGFrntAxl  b=PlntVehDstCGRearAxl  m=PlntVehMass  Cy_f=DriverFrontCornerStiff  Cy_r=DriverRearCornerStiff  I=PlntVehYawMomentInertia  Ksteer=PlntSteerRatio  theta=DriverWheelRange  Idl=1  Re=PlntWhlLdRadius  lambda_mu=1  GearInit=DriverInitialGear  tShift=DriverShiftTime  pdlVec=[0.1 0.4 0.5 0.9]  upShftTbl=[-1 12.9375 26.4375 39.9375 51.18749999999999 62.4375 72.84375 83.25;-1 16.3125 29.8125 43.3125 54.5624 65.8125 76.78125 87.75;-1 19.6875 33.1875 46.68749999999999 57.9375 69.1875 80.71875 92.25;-1 33 52.5 77.25 100.5 138.75 161.875 185]  dwnShftTbl=[-1 12.9375 26.4375 39.9375 51.18749999999999 62.4375 72.84375 83.25;-1 16.3125 29.8125 43.3125 54.5624 65.8125 76.78125 87.75;-1 19.6875 33.1875 46.68749999999999 57.9375 69.1875 80.71875 92.25;-1 33 52.5 77.25 100.5 138.75 161.875 185]  tClutch=.5  tRev=.5  tPark=120  UpGearVec="[0  1  2  3  4  5  6  7]"  DownGearVec="[1  2  3  4  5  6  7  8]"  aMode=2
  Terminator : Terminator
  To Nonvirtual Bus : SignalConversion  ConversionOutput=Virtual bus  OverrideOpt=off
  Unit Conversion : UnitConversion
  VVCLightsCmd : Constant  Value=0  OutDataTypeStr=Bus: VVCLightsCmdBUS  SampleTime=-1
  Driver : Outport  VectorParamsAs1DForOutWhenUnconnected=off
  wires:
  Bus Selector1/14 -> Hill Hold & Stop/5(<DecelZero>)  "<DecelZero>"
  To Nonvirtual Bus/1 -> Bus Creator1/6  "LightsCmd"
  VVCLightsCmd/1 -> To Nonvirtual Bus/1
  Unit Conversion/1 -> Linear Predictive Driver/1, Hill Hold & Stop/1(LngRef)
  Hill Hold & Stop/1(EnblDecelOvr) -> Linear Predictive Driver/11
  Hill Hold & Stop/2(DecelOvrCmd) -> Linear Predictive Driver/12
  Hill Hold & Stop/3(DecelHld) -> Linear Predictive Driver/13
  Hill Hold & Stop/4(DecelZero) -> Linear Predictive Driver/14
  Hill Hold & Stop/6(VelFdbk) -> Linear Predictive Driver/16
  Hill Hold & Stop/5(Grade) -> Linear Predictive Driver/15
  Env/1 -> Hill Hold & Stop/6(Env)
  Bus Selector1/13 -> Hill Hold & Stop/4(<DecelHld>)  "<DecelHld>"
  Bus Selector1/12 -> Hill Hold & Stop/3(<DecelOvrCmd>)  "<DecelCmd>"
  Bus Selector1/11 -> Hill Hold & Stop/2(<EnblDecelCmd>)  "<EnblDecelCmd>"
  Bus Selector1/9 -> Linear Predictive Driver/9  "<AccelHld>"
  Bus Selector1/8 -> Linear Predictive Driver/8  "<AccelCmd>"
  Bus Selector1/7 -> Linear Predictive Driver/7  "<EnblAccelCmd>"
  Bus Selector1/6 -> Linear Predictive Driver/6  "<SteerZero>"
  Bus Selector1/5 -> Linear Predictive Driver/5  "<SteerHld>"
  Bus Selector1/4 -> Linear Predictive Driver/4  "<SteerCmd>"
  Bus Selector1/3 -> Linear Predictive Driver/3  "<EnblSteerCmd>"
  Constant/1 -> Bus Creator1/5  "IgnSwtch"
  Linear Predictive Driver/5 -> Bus Creator1/4  "GearCmd"
  Linear Predictive Driver/4 -> Bus Creator1/3  "DecelCmd"
  Linear Predictive Driver/2 -> Bus Creator1/1  "SteerCmd"
  Bus Selector1/1 -> Unit Conversion/1  "<LngRef>"
  VehRef/1 -> Bus Selector1/1
  Bus Selector/4 -> Linear Predictive Driver/20  "<r>"
  Bus Selector1/2 -> Linear Predictive Driver/2  "<LtrRef>"
  VehFdbk/1 -> Bus Selector/1, Hill Hold & Stop/7(VehFdbk)
  Bus Selector/3 -> Linear Predictive Driver/19  "<psi>"
  Linear Predictive Driver/1 -> Terminator/1
  Bus Creator1/1 -> Driver/1
  Bus Selector1/10 -> Linear Predictive Driver/10  "<AccelZero>"
  Bus Selector/1 -> Linear Predictive Driver/17  "<Y>"
  Linear Predictive Driver/3 -> Bus Creator1/2  "AccelCmd"
  Bus Selector/2 -> Linear Predictive Driver/18  "<Ydot>"

== system ConfiguredVirtualVehicleModelyaris/Driver Commands/Driver Commands/Predictive Stanley Driver ==
  VehRef : Inport
  VehFdbk : Inport  Port=2
  Env : Inport  Port=3
  Bus Creator1 : BusCreator  Inputs=6
  Bus Selector : BusSelector  OutputSignals=Body.InertFrm.Cg.Disp.X,Body.InertFrm.Cg.Disp.Y,Body.InertFrm.Cg.Ang.psi,Body.BdyFrm.Cg.AngVel.r
  Bus Selector1 : BusSelector  OutputSignals=DrvRef.LngRef,DrvRef.XRef,DrvRef.YRef,DrvRef.PhiRef,DrvCmd.SteerCmd.EnblSteerCmd,DrvCmd.SteerCmd.SteerCmd,DrvCmd.SteerCmd.SteerHld,DrvCmd.SteerCmd.SteerZero,DrvCmd.AccelCmd.EnblAccelCmd,DrvCmd.AccelCmd.AccelCmd,DrvCmd.AccelCmd.AccelHld,DrvCmd.AccelCmd.AccelZero,DrvCmd.DecelCmd.EnblDecelCmd,DrvCmd.DecelCmd.DecelCmd,DrvCmd.DecelCmd.DecelHld,DrvCmd.DecelCmd.DecelZero,DrvRef.CurvRef
  Constant : Constant  Value=false
  Hill Hold & Stop : Subsystem
  Linear Predictive Driver : vehdynlibdriver/Predictive Driver  extAccelOvr=on  extDecelOvr=on  extAccelHld=on  extDecelHld=on  extAccelZero=on  extDecelZero=on  extSteerOvr=on  extSteerHld=on  extSteerZero=on  cntrlType=Predictive  cntrlTypeLat=Stanley  shftType=Reverse, Neutral, Drive  coordMode=SAE J670 (Z-down)  refType=Reference pose  velUnits=m/s  angUnits=rad  gearOut=on  steerOut=on  Kp=3  Ki=1  Kff=1  Kg=0  VehVelVec=[0 100]  KffVec=[.1 .1]  KpVec=[10 10]  KiVec=[5 5]  KgVec=[0 0]  vnom=5  Kaw=1  tauerr=.075  tau=DriverTimeConst  L=DriverPreviewDist  Kpt=DriverTractiveForce  aR=DriverRollRes  bR=DriverDrivelineRes  cR=DriverAeroRes  g=EnvGrvty  vecPose=off  dynamMode=on  PositionGainF=DriverPositionGainF  PositionGainR=DriverPositionGainR  YawRateGain=DriverYawRateGain  DelayGain=DriverDelayGain  enableDrift=off  BetaRef=10  KpBeta=1  KpDrift=1  KdDrift=1  KpPsi=1  KOmega=.1  tOmega=.1  a=PlntVehDstCGFrntAxl  b=PlntVehDstCGRearAxl  m=PlntVehMass  Cy_f=DriverFrontCornerStiff  Cy_r=DriverRearCornerStiff  I=PlntVehYawMomentInertia  Ksteer=PlntSteerRatio  theta=DriverWheelRange  Idl=1  Re=PlntWhlLdRadius  lambda_mu=1  GearInit=DriverInitialGear  tShift=DriverShiftTime  pdlVec=[0.1 0.4 0.5 0.9]  upShftTbl=[-1 12.9375 26.4375 39.9375 51.18749999999999 62.4375 72.84375 83.25;-1 16.3125 29.8125 43.3125 54.5624 65.8125 76.78125 87.75;-1 19.6875 33.1875 46.68749999999999 57.9375 69.1875 80.71875 92.25;-1 33 52.5 77.25 100.5 138.75 161.875 185]  dwnShftTbl=[-1 12.9375 26.4375 39.9375 51.18749999999999 62.4375 72.84375 83.25;-1 16.3125 29.8125 43.3125 54.5624 65.8125 76.78125 87.75;-1 19.6875 33.1875 46.68749999999999 57.9375 69.1875 80.71875 92.25;-1 33 52.5 77.25 100.5 138.75 161.875 185]  tClutch=.5  tRev=.5  tPark=120  UpGearVec="[0  1  2  3  4  5  6  7]"  DownGearVec="[1  2  3  4  5  6  7  8]"  aMode=2
  Terminator : Terminator
  To Nonvirtual Bus : SignalConversion  ConversionOutput=Virtual bus  OverrideOpt=off
  Unit Conversion : UnitConversion
  VVCLightsCmd : Constant  Value=0  OutDataTypeStr=Bus: VVCLightsCmdBUS  SampleTime=-1
  Driver : Outport  VectorParamsAs1DForOutWhenUnconnected=off
  wires:
  Bus Selector1/13 -> Hill Hold & Stop/2(<EnblDecelCmd>)  "<EnblDecelCmd>"
  Bus Selector1/14 -> Hill Hold & Stop/3(<DecelOvrCmd>)  "<DecelCmd>"
  Bus Selector1/15 -> Hill Hold & Stop/4(<DecelHld>)  "<DecelHld>"
  Bus Selector1/16 -> Hill Hold & Stop/5(<DecelZero>)  "<DecelZero>"
  Bus Selector1/17 -> Hill Hold & Stop/6(<CurvRef>)  "<CurvRef>"
  Bus Selector1/12 -> Linear Predictive Driver/12  "<AccelZero>"
  Bus Selector/1 -> Linear Predictive Driver/20  "<X>"
  Bus Selector/2 -> Linear Predictive Driver/21  "<Y>"
  Bus Selector/3 -> Linear Predictive Driver/22  "<psi>"
  Bus Selector1/2 -> Linear Predictive Driver/2  "<XRef>"
  Bus Selector1/3 -> Linear Predictive Driver/3  "<YRef>"
  Bus Selector1/4 -> Linear Predictive Driver/4  "<PhiRef>"
  Bus Selector1/5 -> Linear Predictive Driver/5  "<EnblSteerCmd>"
  Bus Selector1/10 -> Linear Predictive Driver/10  "<AccelCmd>"
  Bus Selector1/6 -> Linear Predictive Driver/6  "<SteerCmd>"
  Bus Selector1/9 -> Linear Predictive Driver/9  "<EnblAccelCmd>"
  Bus Selector1/7 -> Linear Predictive Driver/7  "<SteerHld>"
  Bus Selector1/8 -> Linear Predictive Driver/8  "<SteerZero>"
  To Nonvirtual Bus/1 -> Bus Creator1/6  "LightsCmd"
  VVCLightsCmd/1 -> To Nonvirtual Bus/1
  Hill Hold & Stop/6(CurvRef) -> Linear Predictive Driver/18
  Hill Hold & Stop/5(Grade) -> Linear Predictive Driver/17
  Bus Selector/4 -> Linear Predictive Driver/23  "<r>"
  Linear Predictive Driver/3 -> Bus Creator1/2  "AccelCmd"
  Bus Creator1/1 -> Driver/1
  Linear Predictive Driver/1 -> Terminator/1
  VehFdbk/1 -> Bus Selector/1, Hill Hold & Stop/8(VehFdbk)
  VehRef/1 -> Bus Selector1/1
  Bus Selector1/1 -> Unit Conversion/1  "<LngRef>"
  Linear Predictive Driver/2 -> Bus Creator1/1  "SteerCmd"
  Linear Predictive Driver/4 -> Bus Creator1/3  "DecelCmd"
  Linear Predictive Driver/5 -> Bus Creator1/4  "GearCmd"
  Constant/1 -> Bus Creator1/5  "IgnSwtch"
  Bus Selector1/11 -> Linear Predictive Driver/11  "<AccelHld>"
  Env/1 -> Hill Hold & Stop/7(Env)
  Hill Hold & Stop/7(VelFdbk) -> Linear Predictive Driver/19
  Hill Hold & Stop/4(DecelZero) -> Linear Predictive Driver/16
  Hill Hold & Stop/3(DecelHld) -> Linear Predictive Driver/15
  Hill Hold & Stop/2(DecelOvrCmd) -> Linear Predictive Driver/14
  Hill Hold & Stop/1(EnblDecelOvr) -> Linear Predictive Driver/13
  Unit Conversion/1 -> Linear Predictive Driver/1, Hill Hold & Stop/1(LngRef)

== system ConfiguredVirtualVehicleModelyaris/Environment/Ground Feedback/3D Engine ==
  WheelFdbk : Inport
  3D Engine Source : Subsystem  Variant=on  VariantControl=Choice  mask(Terrain Source){terrType=Single point}
      mask prompts: terrType "Terrain feedback type:"
      mask help:
      | This variant subsystem provides the option for:
      | - a single point of contact for each wheel with minimal post-processing ideal for smooth surfaces and maximum run-time performance.
      | - multiple points of contact per wheel which may be used when interested in non-smooth terrain at a higher computational cost and requires Vehicle Dynamics Blockset.
      mask TypeOptions terrType: Single point | Multiple points
  Z : Outport  VectorParamsAs1DForOutWhenUnconnected=off
  DCM : Outport  Port=2  VectorParamsAs1DForOutWhenUnconnected=off
  wires:
  WheelFdbk/1 -> 3D Engine Source/1(WheelFdbk)
  3D Engine Source/1(z) -> Z/1
  3D Engine Source/2(DCM) -> DCM/1

== system ConfiguredVirtualVehicleModelyaris/Environment/Ground Feedback/Constant ==
  Bus Creator : BusCreator  Inputs=4
  Constant1 : Constant  Value=zeros(4,1)
  Constant2 : Constant  Value=repmat(eye(3),1,1,4)  SampleTime=-1
  Demux : Demux
  Signal Specification : SignalSpecification  Unit=m
  Z : Outport  VectorParamsAs1DForOutWhenUnconnected=off
  DCM : Outport  Port=2  VectorParamsAs1DForOutWhenUnconnected=off
  wires:
  Constant1/1 -> Signal Specification/1
  Signal Specification/1 -> Demux/1
  Demux/4 -> Bus Creator/4  "G_RR_z"
  Demux/1 -> Bus Creator/1  "G_FL_z"
  Demux/3 -> Bus Creator/3  "G_RL_z"
  Demux/2 -> Bus Creator/2  "G_FR_z"
  Bus Creator/1 -> Z/1  "z"
  Constant2/1 -> DCM/1  "DCM"

== system ConfiguredVirtualVehicleModelyaris/Environment/Ground Feedback/Height Map ==
  InertFrm : Inport
  "2D Lookup Tbl for Elevation, Z" : Subsystem  TreatAsAtomicUnit=on
      mask init:
      | [~]=vehdynicon('vehdynblk',gcb);
  Bus Creator : BusCreator  Inputs=4
  Bus Selector : BusSelector  OutputSignals=FrntAxl.Lft.Disp.X,FrntAxl.Rght.Disp.X,RearAxl.Lft.Disp.X,RearAxl.Rght.Disp.X
  Bus Selector1 : BusSelector  OutputSignals=FrntAxl.Lft.Disp.Y,FrntAxl.Rght.Disp.Y,RearAxl.Lft.Disp.Y,RearAxl.Rght.Disp.Y
  Constant2 : Constant  Value=repmat(eye(3),1,1,4)  SampleTime=-1
  Demux : Demux
  Signal Specification : SignalSpecification  Unit=m
  Wheel Coordinates : Subsystem
  Z : Outport
  DCM : Outport  Port=2
  wires:
  "2D Lookup Tbl for Elevation, Z"/1(Z) -> Signal Specification/1
  Bus Selector1/4 -> Wheel Coordinates/8(RearAxlRghtY)  "<Y>"
  Bus Selector1/3 -> Wheel Coordinates/7(RearAxlLftY)  "<Y>"
  Bus Selector/1 -> Wheel Coordinates/1(FrntAxlLftX)  "<X>"
  Bus Selector/2 -> Wheel Coordinates/2(FrntAxlRghtX)  "<X>"
  Bus Selector1/2 -> Wheel Coordinates/6(FrntAxlRghtY)  "<Y>"
  Bus Selector/4 -> Wheel Coordinates/4(RearAxlRghtX)  "<X>"
  Bus Selector/3 -> Wheel Coordinates/3(RearAxlLftX)  "<X>"
  Bus Selector1/1 -> Wheel Coordinates/5(FrntAxlLftY)  "<Y>"
  Wheel Coordinates/2(YWhl) -> "2D Lookup Tbl for Elevation, Z"/2(YWhl)
  Wheel Coordinates/1(XWhl) -> "2D Lookup Tbl for Elevation, Z"/1(XWhl)
  InertFrm/1 -> Bus Selector1/1, Bus Selector/1
  Demux/2 -> Bus Creator/2  "G_FR_z"
  Demux/1 -> Bus Creator/1  "G_FL_z"
  Demux/4 -> Bus Creator/4  "G_RR_z"
  Demux/3 -> Bus Creator/3  "G_RL_z"
  Bus Creator/1 -> Z/1  "z"
  Signal Specification/1 -> Demux/1
  Constant2/1 -> DCM/1  "DCM"

== system ConfiguredVirtualVehicleModelyaris/Environment/Ground Feedback/Ideal Inclined Plane ==
  InertFrm : Inport
  Bus Creator : BusCreator  Inputs=4
  Bus Selector : BusSelector  OutputSignals=FrntAxl.Lft.Disp.X,FrntAxl.Rght.Disp.X,RearAxl.Lft.Disp.X,RearAxl.Rght.Disp.X
  Bus Selector1 : BusSelector  OutputSignals=FrntAxl.Lft.Disp.Y,FrntAxl.Rght.Disp.Y,RearAxl.Lft.Disp.Y,RearAxl.Rght.Disp.Y
  Demux : Demux
  Ideal Inclined Plane : Subsystem  mask(Ideal Plane Elevation Generator){phi_o=0, theta_o=0, Z_o=0, psi_o=-PlntVehInitYawAng, phi_est=0, theta_est=0, Z_est=5, plane3D=off, planeX=200, planeY=200}
      mask prompts: phi_o "Initial plane bank angle (about global X axis) [rad]:"; theta_o "Initial plane pitch angle (about global Y axis)  [rad]:"; Z_o "Initial plane elevation (at [0,0,0]) [m]"; psi_o "Initial vehicle yaw angle (about global Z axis) [rad]:"; phi_est "Estimated initial vehicle roll angle [rad]:"; theta_est "Estimated initial vehicle pitch angle [rad]:"; Z_est "Estimated initial vehicle elevation [m]"; plane3D "Enable 3D visualization of plane. Requires the Simulink 3D Animation and the 3D visualization enabled (in the Visualization subsystem). The Empty Scene is recommended when activated."; planeX "Total plane length (in X dimension) [m]:"; planeY "Total plane width (in Y dimension) [m]:"
      mask help:
      | This block accepts time varying bank and pitch angles for an idealized planar surface centered at the global origin (Z+up).
      | The plane roll or bank angle, phi, is about the X axis and pitch angle, theta (negative grade), is about the Y axis.
      | A static vertical offset, Z_o, is also permited.
      | Based on the initial plane angles and vertical offset and vehicle pose, estimates of the initial vehicle roll and pitch are calculated (in the vehicle Z+ down frame). These values can be optionally used to udpate the sldds.
      | Caution should be used to esnure the input signals and initial parameters are consistent at initialzation time.
      | If Simulink 3D Animation is available, the visualization will also include a planar checkerboard surface (changing the default scene may be desired in the Visualization subsystem).
      mask init:
      | vehdynicon('vehdynlibzplane',gcb,0,[]);
      mask Callback plane3D: vehdynicon('vehdynlibzplane',gcb,1,[]);
      mask DialogControl initParams Prompt: Setup Parameters
      mask DialogControl slddUpdate Prompt: Vehicle Pose Estimates
      mask DialogControl updateSLDD Prompt: Update data dictionary with initial roll, pitch and yaw estimates
      mask DialogControl updateSLDD Callback: vehdynicon('vehdynlibzplane',gcb,2,'VirtualVehicleTemplate.sldd');
      mask DialogControl sim3d Prompt: Visualization Options
  Rate Limiter : RateLimiter  RisingSlewLimit=10  FallingSlewLimit=-10  SampleTimeMode=inherited
  Rate Limiter1 : RateLimiter  RisingSlewLimit=10  FallingSlewLimit=-10  SampleTimeMode=inherited
  Signal Specification : SignalSpecification  Unit=m
  Signal Specification1 : SignalSpecification  Unit=deg
  Signal Specification2 : SignalSpecification  Unit=deg
  Slider : SliderBlock  ScaleMin=-30  ScaleMax=30
  Slider1 : SliderBlock  ScaleMin=-30  ScaleMax=30
  Unit Conversion : UnitConversion
  Unit Conversion1 : UnitConversion
  Vector Concatenate : Concatenate  NumInputs=4  Mode=Multidimensional array  ConcatenateDimension=3
  Wheel Coordinates : Subsystem
  Z+up : UnaryMinus
  phiPlane : Constant  Value=0
  thetaPlane : Constant  Value=0
  Z : Outport
  DCM : Outport  Port=2
  wires:
  Ideal Inclined Plane/2(DCM) -> Vector Concatenate/1, Vector Concatenate/2, Vector Concatenate/4, Vector Concatenate/3  "DCM"
  Signal Specification/1 -> Demux/1
  Bus Creator/1 -> Z/1  "z"
  Demux/3 -> Bus Creator/3  "G_RL_z"
  Demux/4 -> Bus Creator/4  "G_RR_z"
  Demux/1 -> Bus Creator/1  "G_FL_z"
  Demux/2 -> Bus Creator/2  "G_FR_z"
  InertFrm/1 -> Bus Selector/1, Bus Selector1/1
  Wheel Coordinates/1(XWhl) -> Ideal Inclined Plane/1(X)
  Wheel Coordinates/2(YWhl) -> Z+up/1
  Bus Selector1/1 -> Wheel Coordinates/5(FrntAxlLftY)  "<Y>"
  Bus Selector/3 -> Wheel Coordinates/3(RearAxlLftX)  "<X>"
  Bus Selector/4 -> Wheel Coordinates/4(RearAxlRghtX)  "<X>"
  Bus Selector1/2 -> Wheel Coordinates/6(FrntAxlRghtY)  "<Y>"
  Bus Selector/2 -> Wheel Coordinates/2(FrntAxlRghtX)  "<X>"
  Bus Selector/1 -> Wheel Coordinates/1(FrntAxlLftX)  "<X>"
  Bus Selector1/3 -> Wheel Coordinates/7(RearAxlLftY)  "<Y>"
  Bus Selector1/4 -> Wheel Coordinates/8(RearAxlRghtY)  "<Y>"
  phiPlane/1 -> Rate Limiter/1
  Ideal Inclined Plane/1(Z) -> Signal Specification/1
  thetaPlane/1 -> Rate Limiter1/1
  Z+up/1 -> Ideal Inclined Plane/2(Y)
  Signal Specification2/1 -> Unit Conversion1/1
  Signal Specification1/1 -> Unit Conversion/1
  Unit Conversion1/1 -> Ideal Inclined Plane/3(phi)
  Unit Conversion/1 -> Ideal Inclined Plane/4(theta)
  Vector Concatenate/1 -> DCM/1  "DCM"
  Rate Limiter/1 -> Signal Specification2/1
  Rate Limiter1/1 -> Signal Specification1/1

== system ConfiguredVirtualVehicleModelyaris/Environment/Ground Feedback/Three-Axle Constant ==
  Bus Creator : BusCreator  Inputs=6
  Constant1 : Constant  Value=zeros(6,1)
  Constant2 : Constant  Value=repmat(eye(3),1,1,6)  SampleTime=-1
  Demux : Demux  Outputs=6
  Signal Specification : SignalSpecification  Unit=m
  Z : Outport  VectorParamsAs1DForOutWhenUnconnected=off
  DCM : Outport  Port=2  VectorParamsAs1DForOutWhenUnconnected=off
  wires:
  Demux/4 -> Bus Creator/4  "G_MR_z"
  Constant2/1 -> DCM/1  "DCM"
  Bus Creator/1 -> Z/1  "z"
  Demux/2 -> Bus Creator/2  "G_FR_z"
  Demux/3 -> Bus Creator/3  "G_ML_z"
  Signal Specification/1 -> Demux/1
  Constant1/1 -> Signal Specification/1
  Demux/6 -> Bus Creator/6  "G_RR_z"
  Demux/5 -> Bus Creator/5  "G_RL_z"
  Demux/1 -> Bus Creator/1  "G_FL_z"
